simulink model "Spartan2"  (R2019a)
settings: Solver=FixedStepAuto  StartTime=0.0  StopTime=inf  FixedStep=0.001  RelTol=1e-3
libraries: dspnetwork x1
settings Model: Creator=manuk  LastModifiedBy=manuk
settings DataIOCC: SaveOutput=off  SignalLogging=off  DSMLogging=off  SaveTime=off  ReturnWorkspaceOutputs=off

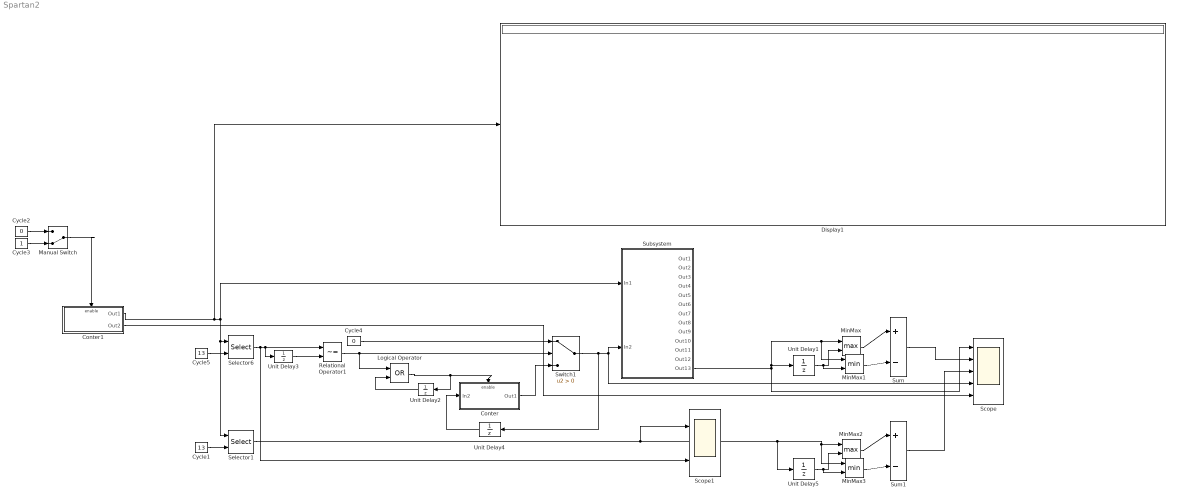
== system Spartan2 ==
  Conter : Subsystem
  Conter1 : Subsystem
  Cycle1 : Constant  Value=13
  Cycle2 : Constant  Value=0
  Cycle3 : Constant
  Cycle4 : Constant  Value=0
  Cycle5 : Constant  Value=13
  Display1 : Display
  Logical Operator : Logic  Operator=OR  AllPortsSameDT=off  OutDataTypeStr=boolean
  Manual Switch : ManualSwitch  CurrentSetting=0
  MinMax : MinMax  Function=max  Inputs=2
  MinMax1 : MinMax  Inputs=2
  MinMax2 : MinMax  Function=max  Inputs=2
  MinMax3 : MinMax  Inputs=2
  Relational Operator1 : RelationalOperator  Operator=~=  OutDataTypeStr=boolean  RndMeth=Simplest
  Scope : Scope  NumInputPorts=5
  Scope1 : Scope  NumInputPorts=2
  Selector1 : Selector  IndexOptions=Index vector (port)  Indices=[6]  OutputSizes=1
  Selector6 : Selector  IndexOptions=Index vector (port)  Indices=[6]  OutputSizes=1
  Subsystem : Subsystem
  Sum : Sum  Inputs=|+-
  Sum1 : Sum  Inputs=|+-
  Switch1 : Switch  Criteria=u2 > Threshold
  Unit Delay1 : UnitDelay  InitialCondition=1  SampleTime=-1  HasFrameUpgradeWarning=on
  Unit Delay2 : UnitDelay  SampleTime=-1  HasFrameUpgradeWarning=on
  Unit Delay3 : UnitDelay  SampleTime=-1  HasFrameUpgradeWarning=on
  Unit Delay4 : UnitDelay  SampleTime=-1  HasFrameUpgradeWarning=on
  Unit Delay5 : UnitDelay  InitialCondition=1  SampleTime=-1  HasFrameUpgradeWarning=on
  wires:
  Conter1/1(Out1) -> Display1/1, Selector1/1, Selector6/1, Subsystem/1(In1)
  Sum/1 -> Scope/2
  MinMax/1 -> Sum/1
  MinMax1/1 -> Sum/2
  Unit Delay1/1 -> MinMax1/2, MinMax/2
  Switch1/1 -> Unit Delay4/1, Scope/4, Subsystem/2(In2)
  Cycle4/1 -> Switch1/1
  Cycle5/1 -> Selector6/2
  Unit Delay3/1 -> Relational Operator1/2
  Relational Operator1/1 -> Logical Operator/1, Switch1/2
  Conter/1(Out1) -> Switch1/3
  Unit Delay2/1 -> Logical Operator/2
  Logical Operator/1 -> Conter/Enable, Unit Delay2/1
  Subsystem/13(Out13) -> MinMax1/1, MinMax/1, Unit Delay1/1, Scope/1
  Unit Delay4/1 -> Conter/1(In2)
  Selector1/1 -> Scope1/1, Unit Delay5/1, MinMax3/1, MinMax2/1
  MinMax3/1 -> Sum1/2
  Unit Delay5/1 -> MinMax3/2, MinMax2/2
  MinMax2/1 -> Sum1/1
  Cycle1/1 -> Selector1/2
  Sum1/1 -> Scope/3
  Cycle2/1 -> Manual Switch/1
  Cycle3/1 -> Manual Switch/2
  Manual Switch/1 -> Conter1/Enable
  Conter1/2(Out2) -> Scope/5
  Selector6/1 -> Scope1/2, Relational Operator1/1, Unit Delay3/1

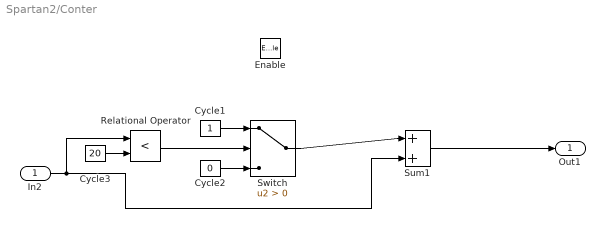
== system Spartan2/Conter ==
  In2 : Inport
  Enable : EnablePort
  Cycle1 : Constant
  Cycle2 : Constant  Value=0
  Cycle3 : Constant  Value=20
  Relational Operator : RelationalOperator  Operator=<  OutDataTypeStr=boolean  RndMeth=Simplest
  Sum1 : Sum  Inputs=|++
  Switch : Switch  Criteria=u2 > Threshold
  Out1 : Outport  InitialOutput=1
  wires:
  Sum1/1 -> Out1/1
  Cycle3/1 -> Relational Operator/2
  Cycle1/1 -> Switch/1
  Cycle2/1 -> Switch/3
  Switch/1 -> Sum1/1
  In2/1 -> Relational Operator/1, Sum1/2
  Relational Operator/1 -> Switch/2

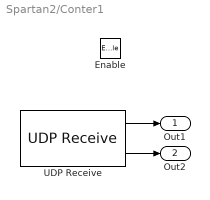
== system Spartan2/Conter1 ==
  Enable : EnablePort
  UDP Receive : dspnetwork/UDP Receive  localURL='0.0.0.0'  localPort=8888  remoteURL='192.168.4.1'  remotePort=-1  recvBufferSize=8192  dims=750  signalDatatype=uint8  isComplex=off  isVarSize=off  showBlockingTime=off  blockingTime=0  sampletime=-1  blockPlatform=[]
      settings: SourceProductName=Simulink
  Out1 : Outport
  Out2 : Outport  Port=2
  wires:
  UDP Receive/1 -> Out1/1
  UDP Receive/2 -> Out2/1

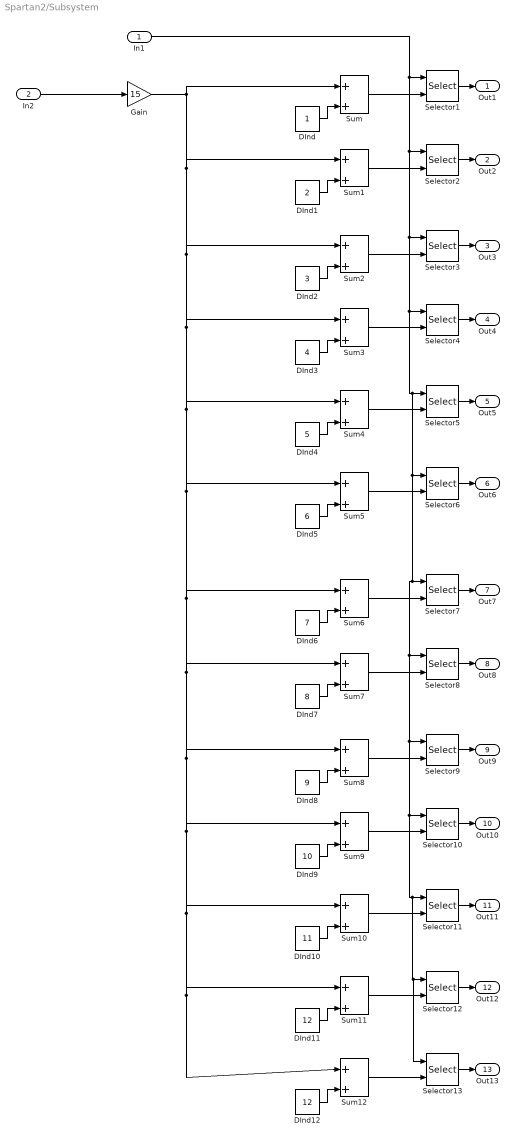
== system Spartan2/Subsystem ==
  In1 : Inport
  In2 : Inport  Port=2
  DInd : Constant
  DInd1 : Constant  Value=2
  DInd10 : Constant  Value=11
  DInd11 : Constant  Value=12
  DInd12 : Constant  Value=12
  DInd2 : Constant  Value=3
  DInd3 : Constant  Value=4
  DInd4 : Constant  Value=5
  DInd5 : Constant  Value=6
  DInd6 : Constant  Value=7
  DInd7 : Constant  Value=8
  DInd8 : Constant  Value=9
  DInd9 : Constant  Value=10
  Gain : Gain  Gain=15
  Selector{1..13} (13 alike) : Selector  IndexOptions=Index vector (port)  Indices=[6]  OutputSizes=1
  Sum{,1..12} (13 alike) : Sum  Inputs=|++
  Out1 : Outport
  Out2 : Outport  Port=2
  Out3 : Outport  Port=3
  Out4 : Outport  Port=4
  Out5 : Outport  Port=5
  Out6 : Outport  Port=6
  Out7 : Outport  Port=7
  Out8 : Outport  Port=8
  Out9 : Outport  Port=9
  Out10 : Outport  Port=10
  Out11 : Outport  Port=11
  Out12 : Outport  Port=12
  Out13 : Outport  Port=13
  wires:
  Sum2/1 -> Selector3/2
  In2/1 -> Gain/1
  DInd1/1 -> Sum1/2
  DInd3/1 -> Sum3/2
  Sum1/1 -> Selector2/2
  Selector3/1 -> Out3/1
  DInd2/1 -> Sum2/2
  DInd4/1 -> Sum4/2
  Sum5/1 -> Selector6/2
  Sum3/1 -> Selector4/2
  DInd5/1 -> Sum5/2
  DInd/1 -> Sum/2
  Sum4/1 -> Selector5/2
  Selector6/1 -> Out6/1
  Sum/1 -> Selector1/2
  Selector5/1 -> Out5/1
  Selector4/1 -> Out4/1
  Selector2/1 -> Out2/1
  Selector1/1 -> Out1/1
  Sum7/1 -> Selector8/2
  Sum8/1 -> Selector9/2
  DInd7/1 -> Sum7/2
  Sum10/1 -> Selector11/2
  Sum9/1 -> Selector10/2
  DInd6/1 -> Sum6/2
  Selector7/1 -> Out7/1
  Selector12/1 -> Out12/1
  Selector9/1 -> Out9/1
  Selector11/1 -> Out11/1
  DInd11/1 -> Sum11/2
  DInd10/1 -> Sum10/2
  Sum11/1 -> Selector12/2
  DInd9/1 -> Sum9/2
  Selector10/1 -> Out10/1
  DInd8/1 -> Sum8/2
  Sum6/1 -> Selector7/2
  Selector8/1 -> Out8/1
  DInd12/1 -> Sum12/2
  Sum12/1 -> Selector13/2
  In1/1 -> Selector13/1, Selector12/1, Selector11/1, Selector10/1, Selector9/1, Selector8/1, Selector7/1, Selector6/1, Selector5/1, Selector4/1, Selector3/1, Selector2/1, Selector1/1
  Selector13/1 -> Out13/1
  Gain/1 -> Sum/1, Sum1/1, Sum2/1, Sum12/1, Sum11/1, Sum10/1, Sum9/1, Sum8/1, Sum7/1, Sum6/1, Sum5/1, Sum4/1, Sum3/1
